simulink model "ModelSimulation"  (R2024b)
settings: Solver=VariableStepAuto  StartTime=0.0  StopTime=5  FixedStep=TSample  RelTol=1e-3
values from neighbouring files (symbols this model uses):
  b = (Km*0.3)/((1750*(2*pi))/60)    (= 0.000180072449898)    [DC_MotorEquation_Encoder_Parameters.m]    (also in DahlinModel_Parameters_Student.m = 0.0003; DeadBeatModel_Parameters_Student.m = 0.0011; dc_motor_data.m = 0.0011)
  J = 0.352e-4    (= 3.52e-05)    [DC_MotorEquation_Encoder_Parameters.m]    (also in DahlinModel_Parameters_Student.m = 7.32e-05; DeadBeatModel_Parameters_Student.m = 0.00010043; dc_motor_data.m = 0.00010043)
  Km = 0.11    [DC_MotorEquation_Encoder_Parameters.m]    (also in DahlinModel_Parameters_Student.m; DeadBeatModel_Parameters_Student.m; dc_motor_data.m)
  Kpi = L/tao_pid_current    (= 6.2)    [dc_motor_data.m]
  Kpw = J/(tao_pid_speed*Km)    (= 0.0913)    [dc_motor_data.m]
  L = 4.1e-3    (= 0.0041)    [DC_MotorEquation_Encoder_Parameters.m]    (also in DahlinModel_Parameters_Student.m; DeadBeatModel_Parameters_Student.m = 0.0062; dc_motor_data.m = 0.0062)
  PulseNumber = 2048*4    (= 8192)    [BaseModelForControl_Parameters.m]    (also in DC_MotorEquation_Encoder_Parameters.m; DahlinModel_Parameters_Student.m; DeadBeatModel_Parameters_Student.m; dc_motor_data.m)
  R = 3.2    [DC_MotorEquation_Encoder_Parameters.m]    (also in DahlinModel_Parameters_Student.m; DeadBeatModel_Parameters_Student.m = 3.2545; dc_motor_data.m = 3.2545)
  RadiantsPerCount = 2*pi/(PulseNumber-1)    (= 0.00076708403213)    [BaseModelForControl_Parameters.m]    (also in DC_MotorEquation_Encoder_Parameters.m; DahlinModel_Parameters_Student.m; DeadBeatModel_Parameters_Student.m; dc_motor_data.m)
  RadToRpm = 60/(2*pi)    (= 9.54929658551)    [BaseModelForControl_Parameters.m]    (also in DC_MotorEquation_Encoder_Parameters.m; DahlinModel_Parameters_Student.m; DeadBeatModel_Parameters_Student.m; dc_motor_data.m)
  RpmToRads = 2*pi/60    (= 0.10471975512)    [BaseModelForControl_Parameters.m]    (also in DC_MotorEquation_Encoder_Parameters.m; DahlinModel_Parameters_Student.m; DeadBeatModel_Parameters_Student.m; dc_motor_data.m)
  TaoFilterOmega = b_filter*TSample/a_filter    (= 0.0009)    [BaseModelForControl_Parameters.m]    (also in DahlinModel_Parameters_Student.m = 0.002; DeadBeatModel_Parameters_Student.m = 0.005; dc_motor_data.m = 0.005)
  Tii = L/R    (= 0.00190505453987)    [dc_motor_data.m]
  Tiw = tao_m    (= 0.0913)    [dc_motor_data.m]
  TSample = PWM_Period    (= 0.0001)    [BaseModelForControl_Parameters.m]    (also in DahlinModel_Parameters_Student.m; DeadBeatModel_Parameters_Student.m; dc_motor_data.m)
undefined symbols (not defined in the file or in its folder): den_Dz_dahlin, DiscIntNeverNeededParam, dspblkCoreblockFVToolHelper, gamma_dahlin, gamma_deadbeat, gcbh, num_Dz_dahlin, num_Dz_deadbeat
libraries: simulink x2
settings Model: Creator=Davide  LastModifiedBy=Utente
settings DataIOCC: ReturnWorkspaceOutputs=off
settings RTWCC: GPUComputeCapability=3.5

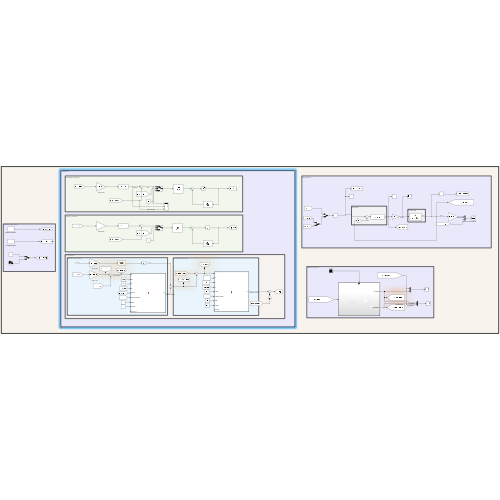
[thumbnail: Simulink's stored preview of the top-level diagram]
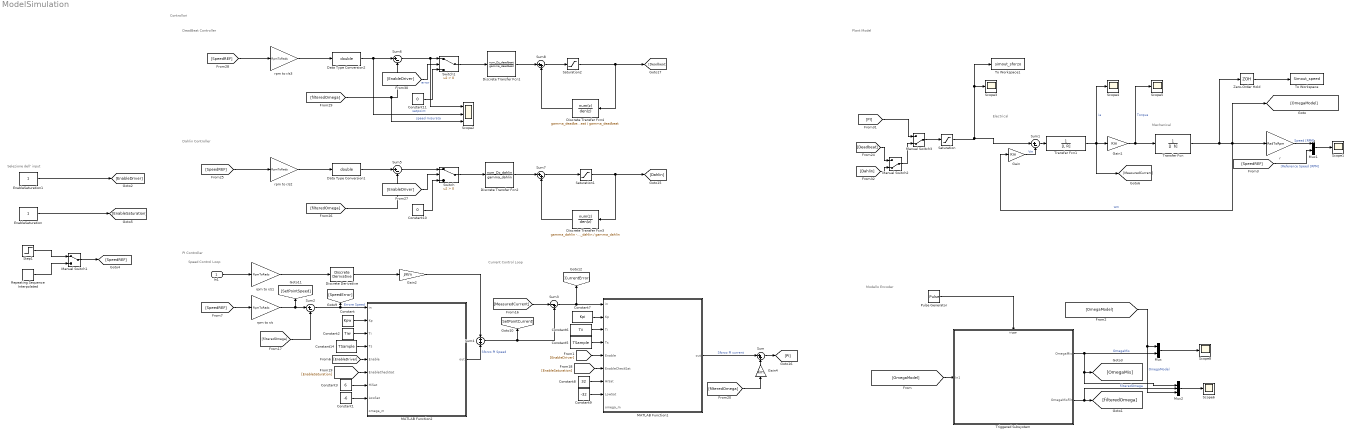
== system ModelSimulation ==
  note: Plant Model
  note: Controllori
  note: Modello Encoder
  note: Mechanical
  note: Electrical
  note: Dahlin Controller
  note: DeadBeat Controller
  note: PI Controller
  note: Speed Control Loop
  note: Current Control Loop
  note: Selezione dell' input
  In1 : Inport  OutDataTypeStr=double
  Constant : Constant  Value=Kpw
  Constant1 : Constant  Value=-6
  Constant10 : Constant  Value=0
  Constant11 : Constant  Value=0
  Constant14 : Constant  Value=TSample
  Constant2 : Constant  Value=Tiw
  Constant3 : Constant  Value=6
  Constant5 : Constant  Value=TSample
  Constant6 : Constant  Value=Tii
  Constant7 : Constant  Value=Kpi
  Constant8 : Constant  Value=32
  Constant9 : Constant  Value=-32
  Data Type Conversion1 : DataTypeConversion  OutDataTypeStr=double  SaturateOnIntegerOverflow=off  RndMeth=Floor
  Data Type Conversion2 : DataTypeConversion  OutDataTypeStr=double  SaturateOnIntegerOverflow=off  RndMeth=Floor
  Discrete Transfer Fcn1 : DiscreteTransferFcn  LoadFcn=dspblkCoreblockFVToolHelper(gcbh,'load');  Numerator=num_Dz_deadbeat  Denominator=gamma_deadbeat
      settings: CopyFcn=dspblkCoreblockFVToolHelper(gcbh,'copy');  DeleteFcn=dspblkCoreblockFVToolHelper(gcbh,'close');  ModelCloseFcn=dspblkCoreblockFVToolHelper(gcbh,'close');  PreSaveFcn=dspblkCoreblockFVToolHelper(gcbh,'presave');  PostSaveFcn=dspblkCoreblockFVToolHelper(gcbh,'postsave');  CloseFcn=dspblkCoreblockFVToolHelper(gcbh,'close');
  Discrete Transfer Fcn2 : DiscreteTransferFcn  LoadFcn=dspblkCoreblockFVToolHelper(gcbh,'load');  Numerator=num_Dz_dahlin  Denominator=gamma_dahlin
      settings: CopyFcn=dspblkCoreblockFVToolHelper(gcbh,'copy');  DeleteFcn=dspblkCoreblockFVToolHelper(gcbh,'close');  ModelCloseFcn=dspblkCoreblockFVToolHelper(gcbh,'close');  PreSaveFcn=dspblkCoreblockFVToolHelper(gcbh,'presave');  PostSaveFcn=dspblkCoreblockFVToolHelper(gcbh,'postsave');  CloseFcn=dspblkCoreblockFVToolHelper(gcbh,'close');
  Discrete Transfer Fcn3 : DiscreteTransferFcn  LoadFcn=dspblkCoreblockFVToolHelper(gcbh,'load');  Numerator="gamma_dahlin -  den_Dz_dahlin"  Denominator=gamma_dahlin
      settings: CopyFcn=dspblkCoreblockFVToolHelper(gcbh,'copy');  DeleteFcn=dspblkCoreblockFVToolHelper(gcbh,'close');  ModelCloseFcn=dspblkCoreblockFVToolHelper(gcbh,'close');  PreSaveFcn=dspblkCoreblockFVToolHelper(gcbh,'presave');  PostSaveFcn=dspblkCoreblockFVToolHelper(gcbh,'postsave');  CloseFcn=dspblkCoreblockFVToolHelper(gcbh,'close');
  Discrete Transfer Fcn4 : DiscreteTransferFcn  LoadFcn=dspblkCoreblockFVToolHelper(gcbh,'load');  Numerator=gamma_deadbeat-den_Dz_deadbeat  Denominator=gamma_deadbeat
      settings: CopyFcn=dspblkCoreblockFVToolHelper(gcbh,'copy');  DeleteFcn=dspblkCoreblockFVToolHelper(gcbh,'close');  ModelCloseFcn=dspblkCoreblockFVToolHelper(gcbh,'close');  PreSaveFcn=dspblkCoreblockFVToolHelper(gcbh,'presave');  PostSaveFcn=dspblkCoreblockFVToolHelper(gcbh,'postsave');  CloseFcn=dspblkCoreblockFVToolHelper(gcbh,'close');
  Discrete Derivative : simulink/Discrete/Discrete Derivative  gainval=1.0  ICPrevScaledInput=0.0  OutMin=[]  OutMax=[]  OutDataType=fixdt(1, 16)  OutScaling=2^-10  DoSatur=off
  EnableSaturation : Constant
  EnableSaturation1 : Constant
  Gain : Gain  Gain=Km
  Gain1 : Gain  Gain=Km
  Gain2 : Gain  Gain=J/Km
  Gain4 : Gain  Gain=Km
  MATLAB Function1 : MATLAB Function  TreatAsAtomicUnit=on
  MATLAB Function2 : MATLAB Function  TreatAsAtomicUnit=on
  Manual Switch1 : ManualSwitch
  Manual Switch2 : ManualSwitch  CurrentSetting=0
  Manual Switch3 : ManualSwitch  CurrentSetting=0
  Mux : Mux  Inputs=2
  Mux1 : Mux  Inputs=2
  Mux2 : Mux  Inputs=3
  Pulse Generator : DiscretePulseGenerator  PulseType=Time based  Period=TSample  PulseWidth=50
  Repeating Sequence Interpolated : simulink/Sources/Repeating Sequence Interpolated  OutValues=[0 800 1000 1000 500 0 0 -500 -500 0].'  TimeValues=[0 0.3 0.5 1 1.2 1.4 1.7 2 2.2 2.5].'  LookUpMeth=Interpolation-Use End Values  tsamp=0.0001  OutMin=[]  OutMax=[]  OutDataTypeStr=double  OutputDataTypeScalingMode=double  OutDataType=fixdt(0,8)  OutScaling=2^-10
  Saturation : Saturate  UpperLimit=32  LowerLimit=-32
  Saturation1 : Saturate  UpperLimit=32  LowerLimit=-32
  Saturation2 : Saturate  UpperLimit=32  LowerLimit=-32
  Scope{1,3..6,8} (6 alike) : Scope
  Scope2 : Scope  NumInputPorts=3
  Step1 : Step  After=100  SampleTime=0
  Sum : Sum  Inputs=|++
  Sum{1..2,5..6} (4 alike) : Sum  Inputs=|+-
  Sum3 : Sum  Inputs=|-+
  Sum4 : Sum  Inputs=+|+
  Sum7 : Sum  Inputs=|++
  Sum8 : Sum  Inputs=|++
  Switch : Switch  Criteria=u2 > Threshold  SaturateOnIntegerOverflow=off  InputSameDT=off
  Switch1 : Switch  Criteria=u2 > Threshold  SaturateOnIntegerOverflow=off  InputSameDT=off
  To Workspace : ToWorkspace  VariableName=Simout_speed  SampleTime=-1
  To Workspace1 : ToWorkspace  VariableName=simout_sforzo  SampleTime=-1
  Transfer Fcn : TransferFcn  Denominator="[J  b]"
  Transfer Fcn1 : TransferFcn  Denominator=[L R]
  Triggered Subsystem : Subsystem  TreatAsAtomicUnit=on
  Zero-Order Hold : ZeroOrderHold  SampleTime=TSample
  "r " : Gain  Gain=RadToRpm  SaturateOnIntegerOverflow=on  OutDataTypeStr=Inherit: Same as input  ParamDataTypeStr=Inherit: Same as input
  rpm to r/s{,1..3} (4 alike) : Gain  Gain=RpmToRads  SaturateOnIntegerOverflow=on  OutDataTypeStr=Inherit: Same as input  ParamDataTypeStr=Inherit: Same as input
  wires:
  Transfer Fcn/1 -> Zero-Order Hold/1, Gain/1, "r "/1, [OmegaModel]  "wm"
  Gain/1 -> Sum1/2  "Vm"
  Gain1/1 -> Scope5/1, Transfer Fcn/1  "Torque"
  Sum1/1 -> Transfer Fcn1/1
  Transfer Fcn1/1 -> Scope4/1, [MeasuredCurrent], Gain1/1  "ia"
  Pulse Generator/1 -> Triggered Subsystem/Trigger
  Mux/1 -> Scope8/1
  Triggered Subsystem/1(OmegaMis) -> Mux2/1, [OmegaMis], Mux/2  "OmegaMis"
  [OmegaModel] -> Triggered Subsystem/1(In1)
  [OmegaModel] -> Mux2/3, Mux/1  "OmegaModel"
  Triggered Subsystem/2(OmegaMisFilt) -> Mux2/2, [filteredOmega]  "filteredOmega"
  Mux1/1 -> Scope1/1
  [SpeedREF] -> Mux1/2  "[Reference Speed [RPM]"
  Mux2/1 -> Scope6/1
  Zero-Order Hold/1 -> To Workspace/1
  [filteredOmega] -> Scope2/3, Sum6/2  "speed misurata"
  Discrete Transfer Fcn4/1 -> Sum8/2
  Sum6/1 -> Scope2/1, Switch1/1  "error"
  Sum/1 -> [PI]
  Manual Switch1/1 -> [SpeedREF]
  [SpeedREF] -> rpm to r/s3/1
  rpm to r/s3/1 -> Data Type Conversion2/1
  Constant11/1 -> Switch1/3
  [EnableDriver] -> Switch1/2
  EnableSaturation/1 -> [EnableSaturation]
  [EnableDriver] -> MATLAB Function1/5(Enable)
  Gain2/1 -> Sum4/1
  [filteredOmega] -> Sum2/2
  Constant10/1 -> Switch/3
  Gain4/1 -> Sum/2
  [EnableSaturation] -> MATLAB Function1/6(EnableCheckSat)
  [MeasuredCurrent] -> Sum3/1
  [filteredOmega] -> Gain4/1
  rpm to r/s2/1 -> Data Type Conversion1/1
  [EnableSaturation] -> MATLAB Function2/6(EnableCheckSat)
  rpm to r/s1/1 -> Discrete Derivative/1
  Saturation1/1 -> Discrete Transfer Fcn3/1, [Dahlin]
  Constant9/1 -> MATLAB Function1/8(LowSat)
  Discrete Derivative/1 -> Gain2/1
  Constant8/1 -> MATLAB Function1/7(HiSat)
  Discrete Transfer Fcn2/1 -> Sum7/1
  Data Type Conversion2/1 -> Scope2/2, Sum6/1  "setpoint"
  Constant6/1 -> MATLAB Function1/3(Ti)
  Sum2/1 -> MATLAB Function2/1(in), [SpeedError]  "Errore Speed"
  [SpeedREF] -> rpm to r/s2/1
  Constant3/1 -> MATLAB Function2/7(HiSat)
  rpm to r/s/1 -> [SetPointSpeed], Sum2/1
  Constant14/1 -> MATLAB Function2/4(Ts)
  Sum4/1 -> Sum3/2, [SetPointCurrent]
  Constant1/1 -> MATLAB Function2/8(LowSat)
  [EnableDriver] -> MATLAB Function2/5(Enable)
  MATLAB Function2/1(out) -> Sum4/2  "Sforzo PI Speed"
  MATLAB Function1/1(out) -> Sum/1  "Sforzo PI current"
  Sum7/1 -> Saturation1/1
  Constant5/1 -> MATLAB Function1/4(Ts)
  EnableSaturation1/1 -> [EnableDriver]
  [SpeedREF] -> rpm to r/s/1
  Sum3/1 -> [CurrentError], MATLAB Function1/1(in)
  [EnableDriver] -> Switch/2
  Discrete Transfer Fcn3/1 -> Sum7/2
  Constant2/1 -> MATLAB Function2/3(Ti)
  Constant/1 -> MATLAB Function2/2(Kp)
  Sum5/1 -> Switch/1
  Constant7/1 -> MATLAB Function1/2(Kp)
  In1/1 -> rpm to r/s1/1
  Data Type Conversion1/1 -> Sum5/1
  [filteredOmega] -> Sum5/2
  Step1/1 -> Manual Switch1/1
  Repeating Sequence Interpolated/1 -> Manual Switch1/2
  [PI] -> Manual Switch3/1
  [Dahlin] -> Manual Switch2/2
  Manual Switch2/1 -> Manual Switch3/2
  [Deadbeat] -> Manual Switch2/1
  "r "/1 -> Mux1/1  "Speed [RPM]"
  Discrete Transfer Fcn1/1 -> Sum8/1
  Sum8/1 -> Saturation2/1
  Manual Switch3/1 -> Saturation/1
  Saturation/1 -> To Workspace1/1, Scope3/1, Sum1/1
  Saturation2/1 -> [Deadbeat], Discrete Transfer Fcn4/1
  Switch1/1 -> Discrete Transfer Fcn1/1
  Switch/1 -> Discrete Transfer Fcn2/1

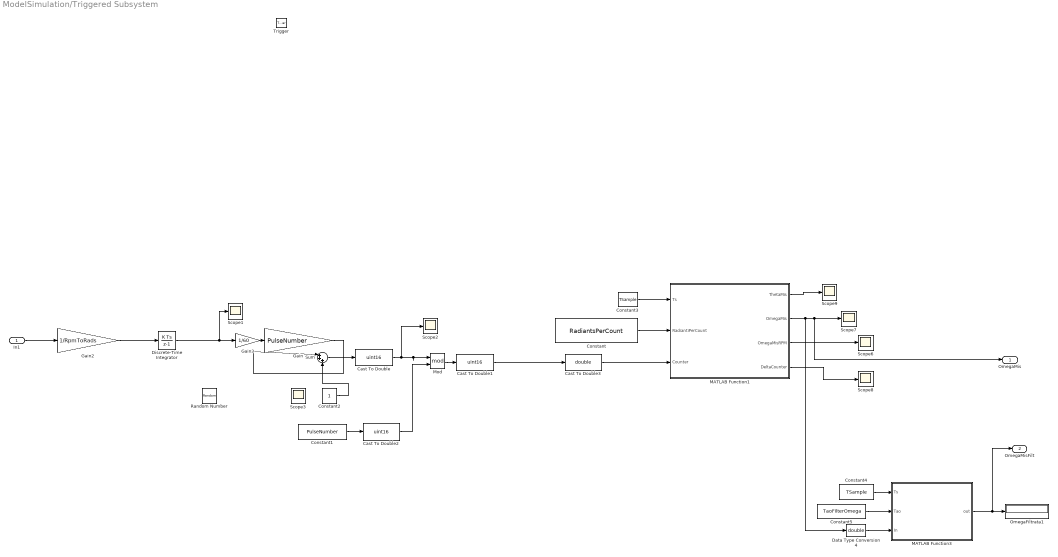
== system ModelSimulation/Triggered Subsystem ==
  In1 : Inport
  Trigger : TriggerPort  VariantControl=(inherit)
  Cast To Double : DataTypeConversion  OutDataTypeStr=uint16  SaturateOnIntegerOverflow=off  RndMeth=Floor
  Cast To Double1 : DataTypeConversion  OutDataTypeStr=uint16  SaturateOnIntegerOverflow=off  RndMeth=Floor
  Cast To Double2 : DataTypeConversion  OutDataTypeStr=uint16  SaturateOnIntegerOverflow=off  RndMeth=Floor
  Cast To Double3 : DataTypeConversion  OutDataTypeStr=double  SaturateOnIntegerOverflow=off  RndMeth=Floor
  Constant : Constant  Value=RadiantsPerCount
  Constant1 : Constant  Value=PulseNumber
  Constant2 : Constant
  Constant3 : Constant  Value=TSample
  Constant4 : Constant  Value=TSample  OutDataTypeStr=double
  Constant5 : Constant  Value=TaoFilterOmega  OutDataTypeStr=double
  Data Type Conversion4 : DataTypeConversion  OutDataTypeStr=double  SaturateOnIntegerOverflow=off  RndMeth=Floor
  Discrete-Time Integrator : DiscreteIntegrator  SampleTime=-1  ICPrevOutput=DiscIntNeverNeededParam  ICPrevScaledInput=DiscIntNeverNeededParam
  Gain : Gain  Gain=PulseNumber
  Gain2 : Gain  Gain=1/RpmToRads
  Gain3 : Gain  Gain=1/60
  MATLAB Function1 : MATLAB Function  TreatAsAtomicUnit=on
  MATLAB Function3 : MATLAB Function  TreatAsAtomicUnit=on
  Mod : Math  Operator=mod
  OmegaFiltrata1 : Display
  Random Number : RandomNumber  Variance=0.3
  Scope{1..3,6..9} (7 alike) : Scope
  Sum : Sum  Inputs=|+++
  OmegaMis : Outport
  OmegaMisFilt : Outport  Port=2
  wires:
  Cast To Double2/1 -> Mod/2
  Cast To Double/1 -> Scope2/1, Mod/1
  Constant1/1 -> Cast To Double2/1
  Mod/1 -> Cast To Double1/1
  Cast To Double1/1 -> Cast To Double3/1
  Gain/1 -> Sum/1
  Constant/1 -> MATLAB Function1/2(RadiantiPerCount)
  Constant3/1 -> MATLAB Function1/1(Ts)
  MATLAB Function1/3(OmegaMisRPM) -> Scope6/1
  Cast To Double3/1 -> MATLAB Function1/3(Counter)
  MATLAB Function1/1(ThetaMis) -> Scope9/1
  MATLAB Function1/2(OmegaMis) -> Data Type Conversion4/1, OmegaMis/1, Scope7/1
  MATLAB Function1/4(DeltaCounter) -> Scope8/1
  Gain3/1 -> Gain/1
  In1/1 -> Gain2/1
  Sum/1 -> Cast To Double/1
  Constant2/1 -> Sum/3
  Data Type Conversion4/1 -> MATLAB Function3/3(In)
  MATLAB Function3/1(out) -> OmegaMisFilt/1, OmegaFiltrata1/1
  Constant5/1 -> MATLAB Function3/2(Tao)
  Constant4/1 -> MATLAB Function3/1(Ts)
  Gain2/1 -> Discrete-Time Integrator/1
  Discrete-Time Integrator/1 -> Scope1/1, Gain3/1

== matlab function ModelSimulation/Triggered Subsystem/MATLAB Function3 ==
  data: Ts input; out output; Tao input; In input
function out  = LowPassFilter(  Ts ,Tao, In)

persistent OutPrecedente
if isempty( OutPrecedente )
    OutPrecedente = 0 ;
end    


    %Filtro passa basso discretizzato con il metodo delle differenze
    %all'indietro
    
    a=Ts/(Ts+Tao);
    b=Tao/(Ts+Tao);
    
    out=a*In+OutPrecedente*b;
   
    OutPrecedente = out;
   
end

== matlab function ModelSimulation/Triggered Subsystem/MATLAB Function1 ==
  data: Ts input; ThetaMis output; RadiantiPerCount input; Counter input; OmegaMis output; OmegaMisRPM output; DeltaCounter output
function [ThetaMis, OmegaMis, OmegaMisRPM, DeltaCounter] = CounterToThetaOmega(Ts, RadiantiPerCount, Counter)

% Inizializzazione dei valori iniziali 
persistent CounterPrec  
if isempty( CounterPrec )
    CounterPrec = 0;
end 

    DeltaCounter=Counter-CounterPrec;
    
    if (DeltaCounter>double(0x1000))
        DeltaCounter=DeltaCounter-double(0x2000);
    end
    
    if (DeltaCounter<-double(0x1000))
        DeltaCounter=DeltaCounter+double(0x2000);
    end
        
    % conversione conteggio in radianti
    ThetaMis = Counter * RadiantiPerCount;
    
    DeltaThetaMis = DeltaCounter*RadiantiPerCount;
   
    OmegaMis = DeltaThetaMis/Ts;
    OmegaMisRPM=OmegaMis*60/(2*pi);
 
    CounterPrec= Counter;
end

== matlab function ModelSimulation/MATLAB Function1 ==
  settings: updateMethod=DISCRETE
  data: in input; out output; Kp input; Ti input; Ts input; Enable input; EnableCheckSat input; HiSat input; LowSat input; omega_m input
function out = PI( in ,Kp , Ti , Ts , Enable, EnableCheckSat, HiSat, LowSat, omega_m)
persistent in_prev out_prev
% Initial Value
if isempty( out_prev )
out_prev = 0;
end
if isempty( in_prev )
in_prev = 0;
end

% G(s)=(Kp/Ti)*((1+Ti*s)/s) (Tustin)
% We run control only if motor is running
if (Enable == 1)
%I Calculate the output
 out = Kp*Ts/(2*Ti)*(in+in_prev) + Kp*(in-in_prev) + out_prev ;
else
out = 0;
in = 0;
end

if(EnableCheckSat == 1)
%check for saturation
if out > HiSat
out = HiSat;
elseif (out < LowSat)
out = LowSat;
end
end

out_prev = out;
in_prev = in;
end

== matlab function ModelSimulation/MATLAB Function2 ==
  settings: updateMethod=DISCRETE
  data: in input; out output; Kp input; Ti input; Ts input; Enable input; EnableCheckSat input; HiSat input; LowSat input; omega_m input
function out = PI( in ,Kp , Ti , Ts , Enable, EnableCheckSat, HiSat, LowSat, omega_m)
persistent in_prev out_prev
% Initial Value
if isempty( out_prev )
out_prev = 0;
end
if isempty( in_prev )
in_prev = 0;
end

% G(s)=(Kp/Ti)*((1+Ti*s)/s) (Tustin)
% We run control only if motor is running
if (Enable == 1)
%I Calculate the output
 out = Kp*Ts/(2*Ti)*(in+in_prev) + Kp*(in-in_prev) + out_prev ;
else
out = 0;
in = 0;
end

if(EnableCheckSat == 1)
%check for saturation
if out > HiSat
out = HiSat;
elseif (out < LowSat)
out = LowSat;
end
end

out_prev = out;
in_prev = in;
end
